simulink model "HydroPowerControlOldV2"  (R2018b)
settings: Solver=FixedStepDiscrete  StartTime=0.0  StopTime=365  FixedStep=1  RelTol=1e-3
values from neighbouring files (symbols this model uses):
  th = 0    [Control_Drift.mat]    (also in Control_Volatillity.mat; main.m)
undefined symbols (not defined in the file or in its folder): DiscIntNeverNeededParam
libraries: simulink x3
settings Model: Creator=h17163  LastModifiedBy=Imrich
settings SFSimCC: SimUseLocalCustomCode=off
settings RTWCC: RTWUseLocalCustomCode=off

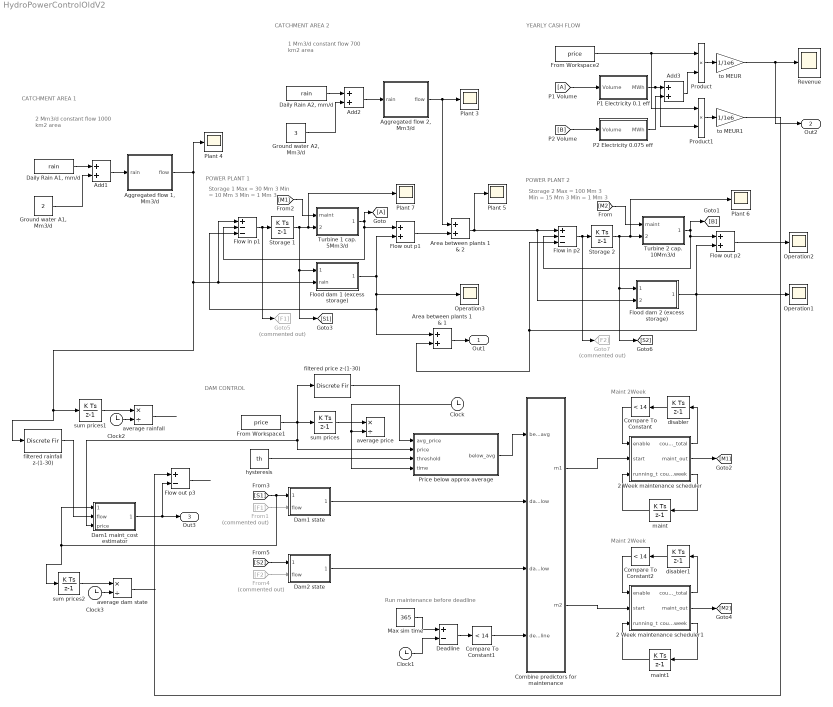
== system HydroPowerControlOldV2 ==
  note: DAM CONTROL
  note: Maint 2Week
  note: Run maintenance before deadline
  note: YEARLY CASH FLOW
  note: 2 Mm3/d constant flow
      | 1000 km2 area
  note: POWER PLANT 1
  note: CATCHMENT AREA 1
  note: Storage 1
      | Max = 30 Mm 3
      | Min = 10 Mm 3
      | Min = 1 Mm 3
  note: Storage 2
      | Max = 100 Mm 3
      | Min = 15 Mm 3
      | Min = 1 Mm 3
  note: POWER PLANT 2
  note: CATCHMENT AREA 2
  note: 1 Mm3/d constant flow
      | 700 km2 area
  note: Maint 2Week
  " disabler" : DiscreteIntegrator  SampleTime=-1  ICPrevOutput=DiscIntNeverNeededParam  ICPrevScaledInput=DiscIntNeverNeededParam
  " disabler1" : DiscreteIntegrator  SampleTime=-1  ICPrevOutput=DiscIntNeverNeededParam  ICPrevScaledInput=DiscIntNeverNeededParam
  2 Week maintenance scheduler : MATLAB Function  TreatAsAtomicUnit=on
  2 Week maintenance scheduler1 : MATLAB Function  TreatAsAtomicUnit=on
  Add1 : Sum
  Add2 : Sum
  Add3 : Sum
  "Aggregated flow 1, Mm3/d" : MATLAB Function  TreatAsAtomicUnit=on
  "Aggregated flow 2, Mm3/d" : MATLAB Function  TreatAsAtomicUnit=on
  Area between plants 1 & 1 : Sum
  Area between plants 1 & 2 : Sum
  Clock{,1..3} (4 alike) : Clock
  Combine predictors for maintenance : MATLAB Function  TreatAsAtomicUnit=on
  Compare To Constant : simulink/Logic and Bit Operations/Compare To Constant  relop=<  const=14  OutDataTypeStr=boolean
  Compare To Constant1 : simulink/Logic and Bit Operations/Compare To Constant  relop=<  const=14  OutDataTypeStr=boolean
  Compare To Constant2 : simulink/Logic and Bit Operations/Compare To Constant  relop=<  const=14  OutDataTypeStr=boolean
  "Daily Rain A1, mm/d" : FromWorkspace  VariableName=rain  SampleTime=0
  "Daily Rain A2, mm/d" : FromWorkspace  VariableName=rain  SampleTime=0
  Dam1 maint_cost estimator : MATLAB Function  TreatAsAtomicUnit=on
  Dam1 state : MATLAB Function  TreatAsAtomicUnit=on
  Dam2 state : MATLAB Function  TreatAsAtomicUnit=on
  Deadline : Sum  Inputs=+-
  Flood dam 1 (excess storage) : MATLAB Function  TreatAsAtomicUnit=on
  Flood dam 2 (excess storage) : MATLAB Function  TreatAsAtomicUnit=on
  Flow in p1 : Sum  Inputs=+--
  Flow in p2 : Sum  Inputs=+--
  Flow out p1 : Sum
  Flow out p2 : Sum
  Flow out p3 : Sum  Inputs=+-
  From Workspace1 : FromWorkspace  VariableName=price  SampleTime=0
  From Workspace2 : FromWorkspace  VariableName=price  SampleTime=0
  From1 : From  Commented=on  GotoTag=F1
  From4 : From  Commented=on  GotoTag=F2
  Goto5 : Goto  Commented=on  GotoTag=F1
  Goto7 : Goto  Commented=on  GotoTag=F2
  "Ground water A1, Mm3/d" : Constant  Value=2
  "Ground water A2, Mm3/d" : Constant  Value=3
  Max sim time : Constant  Value=365
  Operation1 : Scope
  Operation2 : Scope
  Operation3 : Scope
  P1 Electricity 0.1 eff : MATLAB Function  TreatAsAtomicUnit=on
  P2 Electricity 0.075 eff : MATLAB Function  TreatAsAtomicUnit=on
  Plant {3..7} (5 alike) : Scope
  Price below approx average : MATLAB Function  TreatAsAtomicUnit=on
  Product : Product
  Product1 : Product
  Revenue : Scope
  Storage 1 : DiscreteIntegrator  InitialCondition=15  SampleTime=-1  ICPrevOutput=DiscIntNeverNeededParam  ICPrevScaledInput=DiscIntNeverNeededParam
  Storage 2 : DiscreteIntegrator  InitialCondition=50  SampleTime=-1  ICPrevOutput=DiscIntNeverNeededParam  ICPrevScaledInput=DiscIntNeverNeededParam
  Turbine 1 cap. 5Mm3/d : MATLAB Function  TreatAsAtomicUnit=on
  Turbine 2 cap. 10Mm3/d : MATLAB Function  TreatAsAtomicUnit=on
  average dam state : Product  Inputs=*/
  average price : Product  Inputs=*/
  average rainfall : Product  Inputs=*/
  filtered price z-(1-30) : DiscreteFir  Coefficients="[0.0333333333333333\t0.0333333333333333\t0.0333333333333333\t0.0333333333333333\t0.0333333333333333\t0.0333333333333333\t0.0333333333333333\t0.0333333333333333\t0.0333333333333333\t0.0333333333333333\t0.0333333333333333\t0.0333333333333333\t0.0333333333333333\t0.0333333333333333\t0.0333333333333333\t0.0333333333333333\t0.0333333333333333\t0.0333333333333333\t0.0333333333333333\t0.0333333333333333\t0.0333333333333333\t0.0333333333333333\t0.0333333333333333\t0.0333333333333333\t0.0333333333333333\t0.0333333333333333\t0.0333333333333333\t0.0333333333333333\t0.0333333333333333\t0.0333333333333333]"
  filtered rainfall z-(1-30) : DiscreteFir  Coefficients="[0.0333333333333333\t0.0333333333333333\t0.0333333333333333\t0.0333333333333333\t0.0333333333333333\t0.0333333333333333\t0.0333333333333333\t0.0333333333333333\t0.0333333333333333\t0.0333333333333333\t0.0333333333333333\t0.0333333333333333\t0.0333333333333333\t0.0333333333333333\t0.0333333333333333\t0.0333333333333333\t0.0333333333333333\t0.0333333333333333\t0.0333333333333333\t0.0333333333333333\t0.0333333333333333\t0.0333333333333333\t0.0333333333333333\t0.0333333333333333\t0.0333333333333333\t0.0333333333333333\t0.0333333333333333\t0.0333333333333333\t0.0333333333333333\t0.0333333333333333]"
  hysteresis : Constant  Value=th
  maint : DiscreteIntegrator  SampleTime=-1  ICPrevOutput=DiscIntNeverNeededParam  ICPrevScaledInput=DiscIntNeverNeededParam
  maint1 : DiscreteIntegrator  SampleTime=-1  ICPrevOutput=DiscIntNeverNeededParam  ICPrevScaledInput=DiscIntNeverNeededParam
  sum prices : DiscreteIntegrator  SampleTime=-1  ICPrevOutput=DiscIntNeverNeededParam  ICPrevScaledInput=DiscIntNeverNeededParam
  sum prices1 : DiscreteIntegrator  SampleTime=-1  ICPrevOutput=DiscIntNeverNeededParam  ICPrevScaledInput=DiscIntNeverNeededParam
  sum prices2 : DiscreteIntegrator  SampleTime=-1  ICPrevOutput=DiscIntNeverNeededParam  ICPrevScaledInput=DiscIntNeverNeededParam
  to MEUR : Gain  Gain=1/1e6
  to MEUR1 : Gain  Gain=1/1e6
  Out1 : Outport
  Out2 : Outport  Port=2
  Out3 : Outport  Port=3
  wires:
  Add1/1 -> "Aggregated flow 1, Mm3/d"/1(rain)
  Turbine 1 cap. 5Mm3/d/1(output) -> Flow out p1/1, Flow in p1/2, [A]
  Flow in p1/1 -> Goto5/1, Storage 1/1
  Flood dam 1 (excess storage)/1(output) -> Flow in p1/3, Area between plants 1 & 1/1, Operation3/1, Flow out p1/2
  "Daily Rain A1, mm/d"/1 -> Add1/1
  "Ground water A1, Mm3/d"/1 -> Add1/2
  Flood dam 2 (excess storage)/1(output) -> Flow out p2/2, Operation1/1, Area between plants 1 & 1/2, Flow in p2/3
  Area between plants 1 & 2/1 -> Flood dam 2 (excess storage)/2(excess), Flow in p2/1, Plant 5/1
  Flow in p2/1 -> Goto7/1, Storage 2/1
  Turbine 2 cap. 10Mm3/d/1(output) -> Flow out p2/1, Flow in p2/2, [B]
  Storage 2/1 -> Plant 6/1, Turbine 2 cap. 10Mm3/d/2(storage), [S2], Flood dam 2 (excess storage)/1(storage)
  Flow out p2/1 -> Operation2/1
  "Aggregated flow 2, Mm3/d"/1(flow) -> Area between plants 1 & 2/1, Plant 3/1
  "Ground water A2, Mm3/d"/1 -> Add2/2
  "Daily Rain A2, mm/d"/1 -> Add2/1
  Add2/1 -> "Aggregated flow 2, Mm3/d"/1(rain)
  Flow out p1/1 -> Area between plants 1 & 2/2
  Area between plants 1 & 1/1 -> Out1/1
  [M2] -> Turbine 2 cap. 10Mm3/d/1(maint)
  [M1] -> Turbine 1 cap. 5Mm3/d/1(maint)
  [A] -> P1 Electricity 0.1 eff/1(Volume)
  P1 Electricity 0.1 eff/1(MWh) -> Product1/2, Add3/1
  [B] -> P2 Electricity 0.075 eff/1(Volume)
  P2 Electricity 0.075 eff/1(MWh) -> Add3/2
  Add3/1 -> Product/2
  From Workspace2/1 -> Product1/1, Product/1
  Product/1 -> to MEUR/1
  to MEUR/1 -> Revenue/1, Out2/1
  2 Week maintenance scheduler/2(maint_out) -> [M1]
  2 Week maintenance scheduler1/2(maint_out) -> [M2]
  Clock1/1 -> Deadline/2
  maint/1 -> 2 Week maintenance scheduler/3(running_t)
  " disabler"/1 -> Compare To Constant/1
  Max sim time/1 -> Deadline/1
  Deadline/1 -> Compare To Constant1/1
  Compare To Constant1/1 -> Combine predictors for maintenance/4(deadline)
  Compare To Constant/1 -> 2 Week maintenance scheduler/1(enable)
  2 Week maintenance scheduler/1(count_total) -> " disabler"/1
  2 Week maintenance scheduler/3(count_week) -> maint/1
  Combine predictors for maintenance/1(m1) -> 2 Week maintenance scheduler/2(start)
  maint1/1 -> 2 Week maintenance scheduler1/3(running_t)
  2 Week maintenance scheduler1/3(count_week) -> maint1/1
  " disabler1"/1 -> Compare To Constant2/1
  Compare To Constant2/1 -> 2 Week maintenance scheduler1/1(enable)
  2 Week maintenance scheduler1/1(count_total) -> " disabler1"/1
  Combine predictors for maintenance/2(m2) -> 2 Week maintenance scheduler1/2(start)
  Storage 1/1 -> Plant 7/1, Turbine 1 cap. 5Mm3/d/2(storage), [S1], Flood dam 1 (excess storage)/1(storage)
  From1/1 -> Dam1 state/2(flow)
  hysteresis/1 -> Price below approx average/3(threshold)
  Clock/1 -> average price/2, Price below approx average/4(time)
  From Workspace1/1 -> filtered price z-(1-30)/1, Dam1 maint_cost estimator/3(price), Price below approx average/2(price), sum prices/1
  Price below approx average/1(below_avg) -> Combine predictors for maintenance/1(below_avg)
  sum prices/1 -> average price/1
  Dam2 state/1(dam_low) -> Combine predictors for maintenance/3(dam2_low)
  From4/1 -> Dam2 state/2(flow)
  [S2] -> Dam2 state/1(storage)
  Dam1 state/1(dam_low) -> Combine predictors for maintenance/2(dam1_low)
  "Aggregated flow 1, Mm3/d"/1(flow) -> Plant 4/1, sum prices1/1, filtered rainfall z-(1-30)/1, Flow in p1/1, Flood dam 1 (excess storage)/2(rain)
  sum prices1/1 -> average rainfall/1
  Clock2/1 -> average rainfall/2
  Dam1 maint_cost estimator/1(est_maint_cost) -> Flow out p3/2, Out3/1
  filtered price z-(1-30)/1 -> Price below approx average/1(avg_price)
  filtered rainfall z-(1-30)/1 -> Dam1 maint_cost estimator/2(flow)
  average rainfall/1 -> ?
  Product1/1 -> to MEUR1/1
  to MEUR1/1 -> Flow out p3/1
  average dam state/1 -> ?
  Clock3/1 -> average dam state/2
  [S1] -> Dam1 maint_cost estimator/1(storage), sum prices2/1, Dam1 state/1(storage)
  sum prices2/1 -> average dam state/1
  Flow out p3/1 -> ?

== matlab function HydroPowerControlOldV2/Flood dam 1 (excess storage) ==
  data: storage input; output output; rain input
function output = fcn(storage, rain)
if storage >= 30
    output = storage-30+rain;
else
    output = 0;
end

== matlab function HydroPowerControlOldV2/Turbine 1 cap. 5Mm3//d ==
  data: maint input; storage input; output output
function output = fcn(maint, storage)
if storage > 5 & maint == 0
    output = 5;
else
    output = 0;
end

== matlab function HydroPowerControlOldV2/Aggregated flow 1, Mm3//d ==
  data: rain input; flow output
function flow = fcn(rain)
CA1 = 1000; %Catchment area size
flow = (rain/1e3)*(CA1*1e6)/1e6;
end

== matlab function HydroPowerControlOldV2/Flood dam 2 (excess storage) ==
  data: storage input; output output; excess input
function output = fcn(storage, excess)
if storage >= 100
    output = storage-100+excess;
else
    output = 0;
end

== matlab function HydroPowerControlOldV2/Turbine 2 cap. 10Mm3//d ==
  data: maint input; storage input; output output
function output = fcn(maint, storage)
if storage > 10 & maint == 0
    output = 10;
else
    output = 0;
end

== matlab function HydroPowerControlOldV2/Aggregated flow 2, Mm3//d ==
  data: rain input; flow output
function flow = fcn(rain)
CA2 = 700; %Catchment area size
flow = (rain/1e3)*(CA2*1e6)/1e6;
end

== matlab function HydroPowerControlOldV2/P1 Electricity 0.1 eff ==
  data: Volume input; MWh output
function MWh = fcn(Volume)
% 1 ton = 1.25kWh -> 1 kton = 1.25MWh
MWh = Volume*1000*.1;
end

== matlab function HydroPowerControlOldV2/P2 Electricity 0.075 eff ==
  data: Volume input; MWh output
function MWh = fcn(Volume)
% 1 ton = 1.25kWh -> 1 kton = 1.25MWh
MWh = Volume*1000*.075;
end

== matlab function HydroPowerControlOldV2/Price below approx average ==
  data: avg_price input; price input; threshold input; below_avg output; time input
function below_avg = price_watch(avg_price, price, threshold, time)
below_avg=0;

if price+threshold < avg_price && time > 14 %%Wait until average is approximated
    below_avg=1;
end

end

== matlab function HydroPowerControlOldV2/Combine predictors for maintenance ==
  data: below_avg input; dam1_low input; dam2_low input; deadline input; m1 output; m2 output
function [m1,m2] = decision(below_avg, dam1_low, dam2_low, deadline)
m1=0;
m2=0;
if below_avg
    if dam1_low
    	m1=1;
    end
    if dam2_low
        m2=1;
    end
end
    
if deadline
    m1=1;
    m2=1;
end

end

== matlab function HydroPowerControlOldV2/2 Week maintenance scheduler1 ==
  data: enable input; start input; running_t input; count_total output; maint_out output; count_week output
function [count_total, maint_out, count_week] = fc(enable, start, running_t)
%%FC Enables one week of maintenance\
    count_total=0;
    count_week=0;
    maint_out=0;
    
    if enable
        if running_t==0
            if start>0
                count_total=1;
                count_week=1;
                maint_out=1;
            end
            
        elseif running_t < 7 %1-6
            maint_out = 1;
            count_week = 1;
            count_total=1;
            
        elseif running_t >=7
            maint_out = 0;
            count_week = -running_t;
            count_total = 0;
            
            if start > 0 %maintenance immediate restart
                maint_out = 1;
                count_week = -running_t+1;
                count_total = 1;
            end
        end
    end       
end

== matlab function HydroPowerControlOldV2/2 Week maintenance scheduler ==
  data: enable input; start input; running_t input; count_total output; maint_out output; count_week output
function [count_total, maint_out, count_week] = fc(enable, start, running_t)
%%FC Enables one week of maintenance
    count_total=0;
    count_week=0;
    maint_out=0;
    
    if enable
        if running_t==0
            if start>0
                count_total=1;
                count_week=1;
                maint_out=1;
            end
            
        elseif running_t < 7 %1-6
            maint_out = 1;
            count_week = 1;
            count_total=1;
            
        elseif running_t >=7
            maint_out = 0;
            count_week = -running_t;
            count_total = 0;
            
            if start > 0 %maintenance immediate restart
                maint_out = 1;
                count_week = -running_t+1;
                count_total = 1;
            end
        end
    end       
end

== matlab function HydroPowerControlOldV2/Dam1 state ==
  data: storage input; dam_low output; flow input
function dam_low = fcn(storage, flow)
dam_low = 0;
%if flow < 0 && storage < 15
if storage < 10

    dam_low = 1;
end
end

== matlab function HydroPowerControlOldV2/Dam2 state ==
  data: storage input; dam_low output; flow input
function dam_low = fcn(storage, flow)
dam_low = 0;
%if flow < 0 && storage < 50
if storage < 30

    dam_low = 1;
end
end

== matlab function HydroPowerControlOldV2/Dam1 maint_cost estimator ==
  data: storage input; est_maint_cost output; flow input; price input
function est_maint_cost = fcn(storage, flow, price)
dam_max=30;
days=7;
consumption=5;

% Volume to price conversion
MWh = @(Volume) Volume*1000*.1;

% Simulate available volume in dam for next 7 days
sim_stor=storage;
sim_stor_new=sim_stor;
overflow=0;
volume_avail=0;
for i=1:days
    overflow=max(0,sim_stor-dam_max);
    sim_stor_new=sim_stor+flow-overflow;
    
    consumed=min(sim_stor_new,consumption);
    volume_avail=volume_avail+consumed;
    sim_stor=sim_stor_new-consumed;
end

est_maint_cost = price*(MWh(volume_avail))/7;

end
